simulink model "experimentHarnessDLC"  (R2025b)
settings: Solver=VariableStepAuto  StartTime=0.0  StopTime=9.4857  MaxStep=tv.maxSolverStep  RelTol=1e-3
undefined symbols (not defined in the file or in its folder): baseline, scenario
settings Model: Creator=jaiden  LastModifiedBy=r3anjum

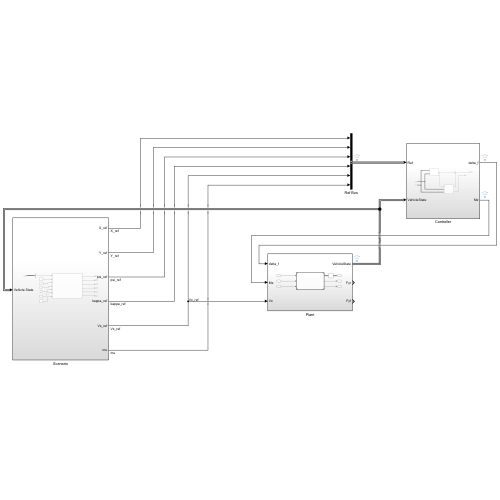
[thumbnail: Simulink's stored preview of the top-level diagram]
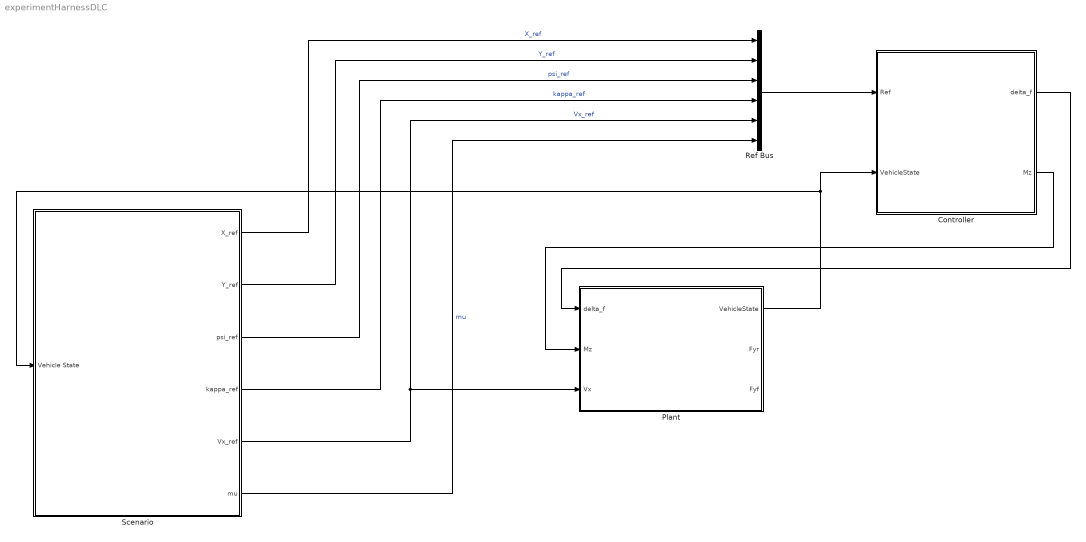
== system experimentHarnessDLC ==
  Controller : Subsystem
  Plant : Subsystem
  Ref Bus : BusCreator  Inputs=6  OutDataTypeStr=Bus: ReferenceBus
  Scenario : Subsystem
  wires:
  Scenario/5(Vx_ref) -> Plant/3(Vx), Ref Bus/5  "Vx_ref"
  Plant/1(VehicleState) -> Scenario/1(Vehicle State), Controller/2(VehicleState)
  Scenario/1(X_ref) -> Ref Bus/1  "X_ref"
  Scenario/2(Y_ref) -> Ref Bus/2  "Y_ref"
  Scenario/3(psi_ref) -> Ref Bus/3  "psi_ref"
  Scenario/4(kappa_ref) -> Ref Bus/4  "kappa_ref"
  Scenario/6(mu) -> Ref Bus/6  "mu"
  Ref Bus/1 -> Controller/1(Ref)
  Controller/1(delta_f) -> Plant/1(delta_f)
  Controller/2(Mz) -> Plant/2(Mz)

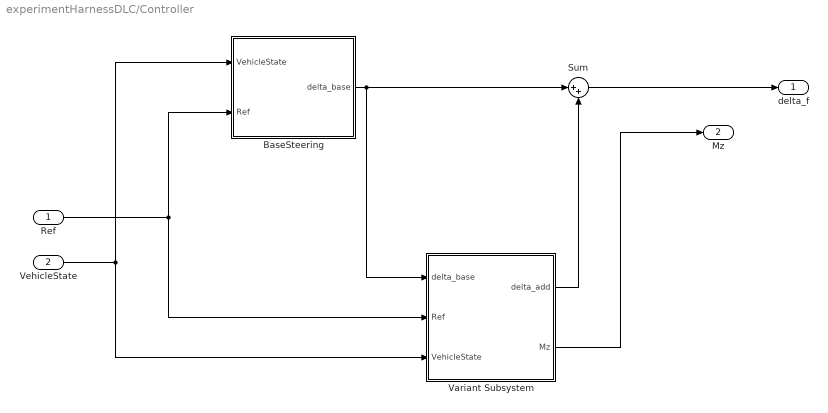
== system experimentHarnessDLC/Controller ==
  Ref : Inport
  VehicleState : Inport  Port=2
  BaseSteering : Subsystem
  Sum : Sum  Inputs=|++
  Variant Subsystem : Subsystem  Variant=on
  delta_f : Outport
  Mz : Outport  Port=2
  wires:
  Ref/1 -> Variant Subsystem/2(Ref), BaseSteering/2(Ref)
  VehicleState/1 -> Variant Subsystem/3(VehicleState), BaseSteering/1(VehicleState)
  BaseSteering/1(delta_base) -> Variant Subsystem/1(delta_base), Sum/1
  Variant Subsystem/1(delta_add) -> Sum/2
  Sum/1 -> delta_f/1
  Variant Subsystem/2(Mz) -> Mz/1

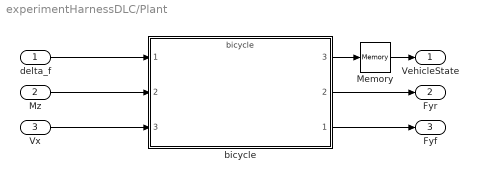
== system experimentHarnessDLC/Plant ==
  delta_f : Inport
  Mz : Inport  Port=2
  Vx : Inport  Port=3
  Memory : Memory
  bicycle : ModelReference  ModelNameDialog=bicycle.slx  SimulationMode=Normal  ModelReferenceVersion=1.9
      settings: PortSchema="{\"entries\":[{\"content\":{\"sides\":[{\"content\":{\"connectorIds\":[\"In1\",\"In2\",\"In3\"]},\"type\":\"ConnectorPlacement.EquallySpacedRectSide\",\"uuid\":\"58d1b5ba-aa94-409a-86bc-1f2a380b806f\"},{\"content\":{\"connectorIds\":[\"Out3\",\"Out2\",\"Out1\"],\"side\":\"RIGHT\"},\"type\":\"ConnectorPlacement.EquallySpacedRectSide\",\"uuid\":\"d4837c49-e6bf-462c-b169-66ee2b0f1817\"},{\"content\":{\"side\":\"TOP\"},\"type\":\"ConnectorPlacement.EquallySpacedRectSide\",\"uuid\":\"4cad5275-f3ab-4015-917f-efe21967d551\"}]},\"type\":\"ConnectorPlacement.EquallySpacedConnector\",\"uuid\":\"b91e3d72-bb0a-4328-b099-f36bf503b2b7\"}],\"packageUris\":[\"http://schema.mathworks.com/mf0/Connector/R2020b\"],\"version\":\"1.0\"}"
  VehicleState : Outport
  Fyr : Outport  Port=2
  Fyf : Outport  Port=3
  wires:
  delta_f/1 -> bicycle/1
  Mz/1 -> bicycle/2
  Vx/1 -> bicycle/3
  bicycle/3 -> Memory/1
  bicycle/2 -> Fyr/1
  bicycle/1 -> Fyf/1
  Memory/1 -> VehicleState/1

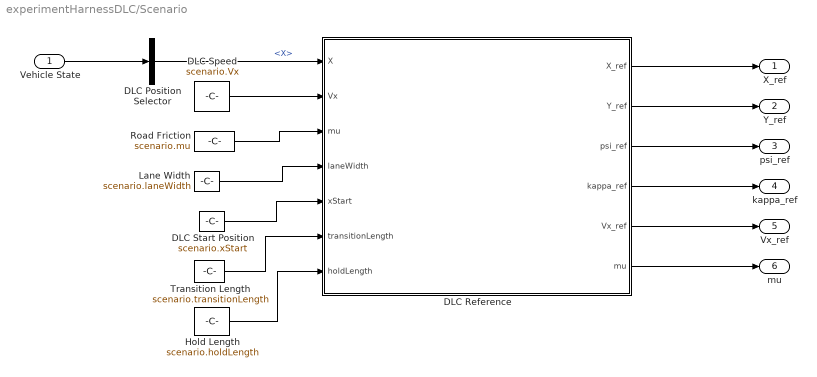
== system experimentHarnessDLC/Scenario ==
  Vehicle State : Inport  OutDataTypeStr=Bus: VehicleStateBus
  DLC Position Selector : BusSelector  OutputSignals=X
  DLC Reference : MATLAB Function  TreatAsAtomicUnit=on
  DLC Speed : Constant  Value=scenario.Vx
  DLC Start Position : Constant  Value=scenario.xStart
  Hold Length : Constant  Value=scenario.holdLength
  Lane Width : Constant  Value=scenario.laneWidth
  Road Friction : Constant  Value=scenario.mu
  Transition Length : Constant  Value=scenario.transitionLength
  X_ref : Outport
  Y_ref : Outport  Port=2
  psi_ref : Outport  Port=3
  kappa_ref : Outport  Port=4
  Vx_ref : Outport  Port=5
  mu : Outport  Port=6
  wires:
  DLC Reference/1(X_ref) -> X_ref/1
  Vehicle State/1 -> DLC Position Selector/1
  DLC Reference/2(Y_ref) -> Y_ref/1
  DLC Reference/3(psi_ref) -> psi_ref/1
  DLC Reference/4(kappa_ref) -> kappa_ref/1
  DLC Reference/5(Vx_ref) -> Vx_ref/1
  DLC Reference/6(mu) -> mu/1
  DLC Speed/1 -> DLC Reference/2(Vx)
  Road Friction/1 -> DLC Reference/3("mu ")
  Lane Width/1 -> DLC Reference/4(laneWidth)
  DLC Start Position/1 -> DLC Reference/5(xStart)
  Transition Length/1 -> DLC Reference/6(transitionLength)
  Hold Length/1 -> DLC Reference/7(holdLength)
  DLC Position Selector/1 -> DLC Reference/1(X)  "<X>"

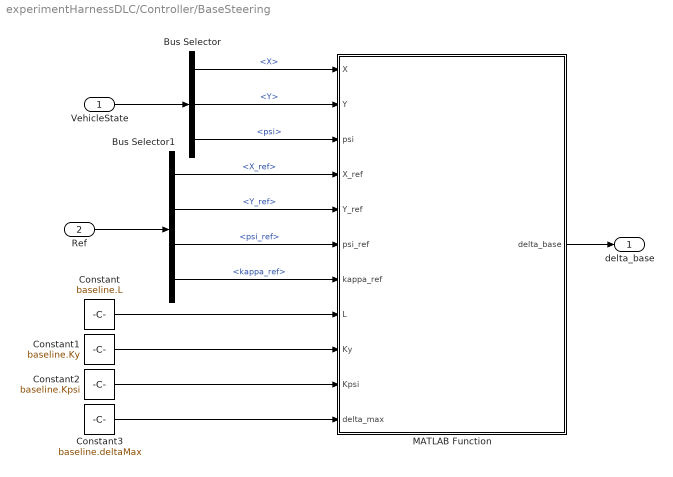
== system experimentHarnessDLC/Controller/BaseSteering ==
  VehicleState : Inport  OutDataTypeStr=Bus: VehicleStateBus
  Ref : Inport  Port=2  OutDataTypeStr=Bus: ReferenceBus
  Bus Selector : BusSelector  OutputSignals=X,Y,psi
  Bus Selector1 : BusSelector  OutputSignals=X_ref,Y_ref,psi_ref,kappa_ref
  Constant : Constant  Value=baseline.L
  Constant1 : Constant  Value=baseline.Ky
  Constant2 : Constant  Value=baseline.Kpsi
  Constant3 : Constant  Value=baseline.deltaMax  VectorParams1D=off
  MATLAB Function : MATLAB Function  TreatAsAtomicUnit=on
  delta_base : Outport
  wires:
  VehicleState/1 -> Bus Selector/1
  Ref/1 -> Bus Selector1/1
  Bus Selector/1 -> MATLAB Function/1(X)  "<X>"
  Bus Selector/2 -> MATLAB Function/2(Y)  "<Y>"
  Bus Selector/3 -> MATLAB Function/3(psi)  "<psi>"
  Bus Selector1/1 -> MATLAB Function/4(X_ref)  "<X_ref>"
  Bus Selector1/2 -> MATLAB Function/5(Y_ref)  "<Y_ref>"
  Bus Selector1/3 -> MATLAB Function/6(psi_ref)  "<psi_ref>"
  Bus Selector1/4 -> MATLAB Function/7(kappa_ref)  "<kappa_ref>"
  Constant/1 -> MATLAB Function/8(L)
  Constant1/1 -> MATLAB Function/9(Ky)
  Constant2/1 -> MATLAB Function/10(Kpsi)
  Constant3/1 -> MATLAB Function/11(delta_max)
  MATLAB Function/1(delta_base) -> delta_base/1

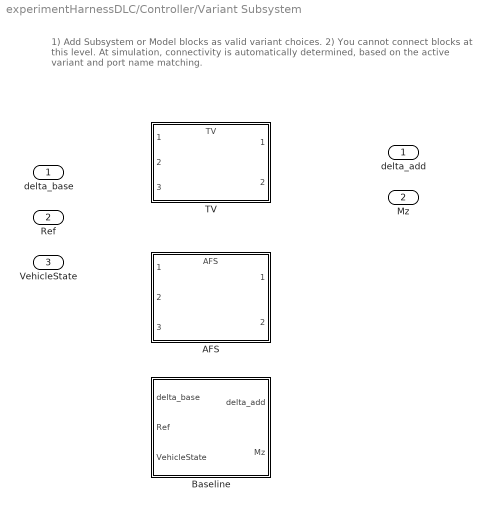
== system experimentHarnessDLC/Controller/Variant Subsystem ==
  note: 1) Add Subsystem or Model blocks as valid variant choices.
      | 2) You cannot connect blocks at this level. At simulation, connectivity is automatically
      | determined, based on the active variant and port name matching.
  delta_base : Inport
  Ref : Inport  Port=2
  VehicleState : Inport  Port=3
  AFS : ModelReference  ModelNameDialog=AFS.slx  SimulationMode=Normal  VariantControl=Choice_1  ModelReferenceVersion=1.10
  Baseline : Subsystem  VariantControl=Choice_2
  TV : ModelReference  ModelNameDialog=TV.slx  SimulationMode=Normal  VariantControl=Choice  ModelReferenceVersion=1.11
  delta_add : Outport
  Mz : Outport  Port=2

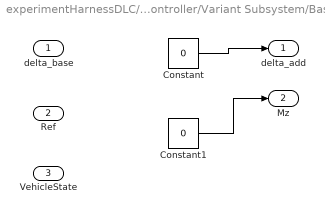
== system experimentHarnessDLC/Controller/Variant Subsystem/Baseline ==
  delta_base : Inport
  Ref : Inport  Port=2  OutDataTypeStr=Bus: ReferenceBus
  VehicleState : Inport  Port=3  OutDataTypeStr=Bus: VehicleStateBus
  Constant : Constant  Value=0
  Constant1 : Constant  Value=0
  delta_add : Outport
  Mz : Outport  Port=2
  wires:
  Constant/1 -> delta_add/1
  Constant1/1 -> Mz/1

== matlab function experimentHarnessDLC/Controller/BaseSteering/MATLAB Function ==
  data: X input; delta_base output; Y input; psi input; X_ref input; Y_ref input; psi_ref input; kappa_ref input; L input; Ky input; Kpsi input; delta_max input
function delta_base = baseSteering( ...
    X, Y, psi, X_ref, Y_ref, psi_ref, kappa_ref, ...
    L, Ky, Kpsi, delta_max)

% Feedforward steering required by the path curvature
delta_ff = atan(L*kappa_ref);

% Signed lateral position error
e_y = -sin(psi_ref)*(X - X_ref) ...
      + cos(psi_ref)*(Y - Y_ref);

% Wrapped heading error in [-pi, pi]
e_psi = atan2(sin(psi_ref - psi), ...
              cos(psi_ref - psi));

% Feedforward plus feedback steering
delta_cmd = delta_ff - Ky*e_y + Kpsi*e_psi;

% Steering-angle limit
delta_base = min(max(delta_cmd, -delta_max), delta_max);

end

== matlab function experimentHarnessDLC/Scenario/DLC Reference ==
  data: X input; X_ref output; Vx input; mu input; laneWidth input; xStart input; transitionLength input; holdLength input; Y_ref output; psi_ref output; kappa_ref output; Vx_ref output; mu output
function [X_ref, Y_ref, psi_ref, kappa_ref, Vx_ref, mu] = ...
    fcn(X, Vx, mu, laneWidth, xStart, transitionLength, holdLength)
%#codegen

[X_ref, Y_ref, psi_ref, kappa_ref, Vx_ref, mu] = ...
    dlcReferenceFromX( ...
    X, ...
    Vx, ...
    mu, ...
    laneWidth, ...
    xStart, ...
    transitionLength, ...
    holdLength);

end
